simulink model "pointEight_Slx"  (R2022b)
settings: Solver=VariableStepAuto  StartTime=0.0  StopTime=10  MaxStep=1e-4  MinStep=1e-5  RelTol=1e-3
settings Model: Creator=yeyi5  LastModifiedBy=yeyi5

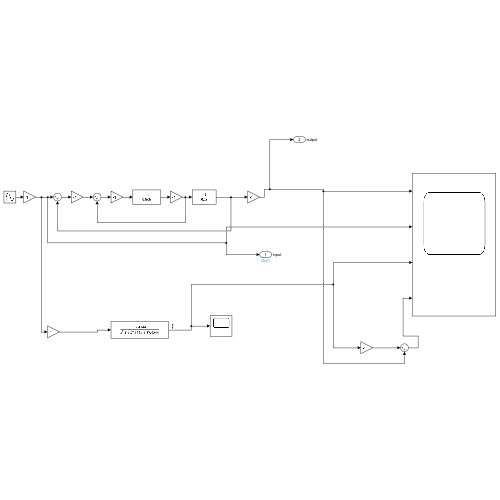
[thumbnail: Simulink's stored preview of the top-level diagram]
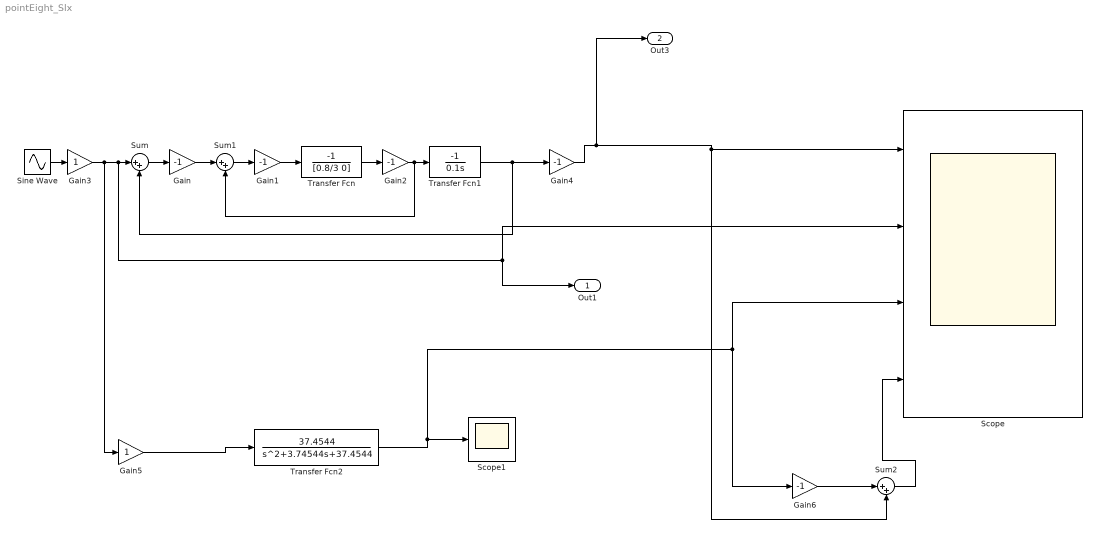
== system pointEight_Slx ==
  Gain{,1..2,4,6} (5 alike) : Gain  Gain=-1
  Gain3 : Gain
  Gain5 : Gain
  Scope : Scope  NumInputPorts=4
  Scope1 : Scope
  Sine Wave : Sin  Amplitude=5  SampleTime=0
  Sum : Sum  Inputs=|++
  Sum1 : Sum  Inputs=|++
  Sum2 : Sum  Inputs=|++
  Transfer Fcn : TransferFcn  Numerator=[-1]  Denominator=[0.8/3 0]
  Transfer Fcn1 : TransferFcn  Numerator=[-1]  Denominator=[0.1 0]
  Transfer Fcn2 : TransferFcn  Numerator=[37.4544]  Denominator=[1 3.74544 37.4544]
  Out1 : Outport  SignalName=input
  Out3 : Outport  Port=2  SignalName=output
  wires:
  Sine Wave/1 -> Gain3/1
  Sum/1 -> Gain/1
  Gain/1 -> Sum1/1
  Sum1/1 -> Gain1/1
  Gain1/1 -> Transfer Fcn/1
  Transfer Fcn/1 -> Gain2/1
  Gain2/1 -> Sum1/2, Transfer Fcn1/1
  Transfer Fcn1/1 -> Sum/2, Gain4/1
  Gain4/1 -> Out3/1, Sum2/2, Scope/1
  Gain5/1 -> Transfer Fcn2/1
  Gain3/1 -> Gain5/1, Out1/1, Scope/2, Sum/1
  Transfer Fcn2/1 -> Gain6/1, Scope/3, Scope1/1
  Gain6/1 -> Sum2/1
  Sum2/1 -> Scope/4
